simulink model "walden_prj_2_5_task1"  (R2025b)
settings: Solver=VariableStepAuto  StartTime=0.0  StopTime=10.0  RelTol=1e-3
settings Model: Creator=nrwal  LastModifiedBy=nrwal

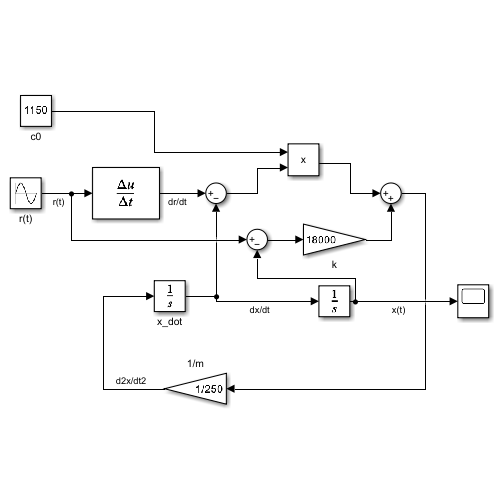
[thumbnail: Simulink's stored preview of the top-level diagram]
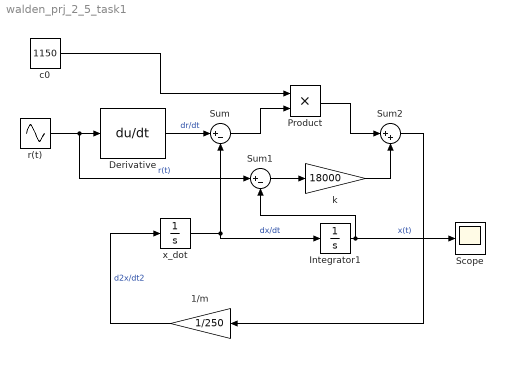
== system walden_prj_2_5_task1 ==
  1/m : Gain  Gain=1/250
  Derivative : Derivative
  Integrator1 : Integrator
  Product : Product
  Scope : Scope
      settings: ActiveDisplayYMinimum=-0.022050663065569576  ActiveDisplayYMaximum=0.021882842453229665
  Sum : Sum  Inputs=|+-
  Sum1 : Sum  Inputs=|+-
  Sum2 : Sum  Inputs=|++
  c0 : Constant  Value=1150
  k : Gain  Gain=18000
  r(t) : Sin  Amplitude=0.01  Frequency=10  SampleTime=0
  x_dot : Integrator
  wires:
  c0/1 -> Product/1
  r(t)/1 -> Sum1/1, Derivative/1  "r(t)"
  Derivative/1 -> Sum/1  "dr/dt"
  Sum/1 -> Product/2
  Sum1/1 -> k/1
  Product/1 -> Sum2/1
  k/1 -> Sum2/2
  Sum2/1 -> 1/m/1
  1/m/1 -> x_dot/1  "d2x/dt2"
  x_dot/1 -> Integrator1/1, Sum/2  "dx/dt"
  Integrator1/1 -> Sum1/2, Scope/1  "x(t)"
